simulink model "task1"  (R2021a)
settings: Solver=FixedStepDiscrete  StartTime=0.0  StopTime=10.0  RelTol=1e-3
libraries: simulink x18
settings Model: Creator=NoteBook  LastModifiedBy=NoteBook
settings OptimizationCC: DefaultParameterBehavior=Inlined  EnhancedBackFolding=on  PassReuseOutputArgsAs=Individual arguments  ZeroExternalMemoryAtStartup=off  ZeroInternalMemoryAtStartup=off  OptimizeBlockOrder=speed  DifferentSizesBufferReuse=on  OptimizationCustomize=off  EfficientTunableParamExpr=on
settings DebuggingCC: ParameterTunabilityLossMsg=error
settings SFSimCC: MATLABDynamicMemAlloc=off
settings RTWCC: SystemTargetFile=ert.tlc  GenCodeOnly=on  TemplateMakefile=ert_default_tmf  GenerateReport=on  LaunchReport=on
settings CodeAppCC: ForceParamTrailComments=on  IgnoreCustomStorageClasses=off  OperatorAnnotations=on  SimulinkDataObjDesc=on  SFDataObjDesc=on  InsertBlockDesc=on
settings ERTTargetCC: TargetLangStandard=C99 (ISO)  GenerateSampleERTMain=on  InlinedParameterPlacement=NonHierarchical  ERTCustomFileTemplate=example_file_process.tlc

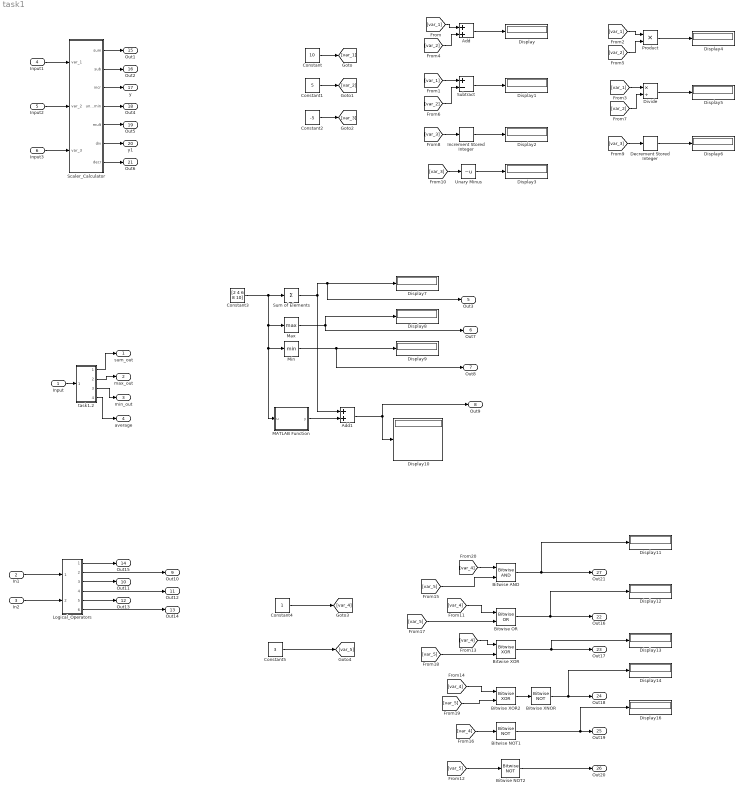
== system task1 ==
  Input : Inport
  In1 : Inport  Port=2
  In2 : Inport  Port=3
  Input1 : Inport  Port=4
  Input2 : Inport  Port=5
  Input3 : Inport  Port=6
  Add : Sum
  Add1 : Sum
  Bitwise AND : simulink/Logic and Bit Operations/Bitwise Operator  logicop=AND  UseBitMask=off  NumInputPorts=2  BitMask=bin2dec('11011001')  BitMaskRealWorld=Stored Integer
  Bitwise NOT1 : simulink/Logic and Bit Operations/Bitwise Operator  logicop=NOT  UseBitMask=off  BitMask=bin2dec('11011001')  BitMaskRealWorld=Stored Integer
  Bitwise NOT2 : simulink/Logic and Bit Operations/Bitwise Operator  logicop=NOT  UseBitMask=off  BitMask=bin2dec('11011001')  BitMaskRealWorld=Stored Integer
  Bitwise OR : simulink/Logic and Bit Operations/Bitwise Operator  logicop=OR  UseBitMask=off  NumInputPorts=2  BitMask=bin2dec('11011001')  BitMaskRealWorld=Stored Integer
  Bitwise XNOR : simulink/Logic and Bit Operations/Bitwise Operator  logicop=NOT  UseBitMask=off  BitMask=bin2dec('11011001')  BitMaskRealWorld=Stored Integer
  Bitwise XOR : simulink/Logic and Bit Operations/Bitwise Operator  logicop=XOR  UseBitMask=off  NumInputPorts=2  BitMask=bin2dec('11011001')  BitMaskRealWorld=Stored Integer
  Bitwise XOR2 : simulink/Logic and Bit Operations/Bitwise Operator  logicop=XOR  UseBitMask=off  NumInputPorts=2  BitMask=bin2dec('11011001')  BitMaskRealWorld=Stored Integer
  Constant : Constant  Value=10
  Constant1 : Constant  Value=5
  Constant2 : Constant  Value=-5
  Constant3 : Constant  Value=[2 4 6 8 10]
  Constant4 : Constant  OutDataTypeStr=uint32
  Constant5 : Constant  Value=3  OutDataTypeStr=uint32
  Decrement Stored Integer : simulink/Additional Math & Discrete/Additional Math: Increment - Decrement/Decrement Stored Integer
      settings: SourceProductBaseCode=SL
  Display{,1..14,16} (16 alike) : Display
  Divide : Product  Inputs=*/
  Increment Stored Integer : simulink/Additional Math & Discrete/Additional Math: Increment - Decrement/Increment Stored Integer
  Logical_Operators : Subsystem
  MATLAB Function : MATLAB Function  TreatAsAtomicUnit=on
  Max : MinMax  Function=max
  Min : MinMax
  Product : Product
  Scaler_Calculator : Subsystem
  Subtract : Sum  Inputs=+-
  Sum of Elements : Sum  Inputs=+
  Unary Minus : UnaryMinus
  task1.2 : Subsystem
  sum_out : Outport
  max_out : Outport  Port=2
  min_out : Outport  Port=3
  average : Outport  Port=4
  Out3 : Outport  Port=5
  Out7 : Outport  Port=6
  Out8 : Outport  Port=7
  Out9 : Outport  Port=8
  Out10 : Outport  Port=9
  Out11 : Outport  Port=10
  Out12 : Outport  Port=11
  Out13 : Outport  Port=12
  Out14 : Outport  Port=13
  Out15 : Outport  Port=14
  Out1 : Outport  Port=15
  Out2 : Outport  Port=16
  y : Outport  Port=17
  Out4 : Outport  Port=18
  Out5 : Outport  Port=19
  y1 : Outport  Port=20
  Out6 : Outport  Port=21
  Out16 : Outport  Port=22
  Out17 : Outport  Port=23
  Out18 : Outport  Port=24
  Out19 : Outport  Port=25
  Out20 : Outport  Port=26
  Out21 : Outport  Port=27
  wires:
  Input/1 -> task1.2/1(In1)
  task1.2/1(Out1) -> sum_out/1
  task1.2/2(Out2) -> max_out/1
  task1.2/3(Out3) -> min_out/1
  task1.2/4(Out4) -> average/1
  Add1/1 -> Out9/1, Display10/1
  Min/1 -> Out8/1, Display9/1
  MATLAB Function/1(y) -> Add1/2
  Max/1 -> Out7/1, Display8/1
  Constant3/1 -> MATLAB Function/1(u), Min/1, Max/1, Sum of Elements/1
  Sum of Elements/1 -> Add1/1, Out3/1, Display7/1
  In1/1 -> Logical_Operators/1(var_1)
  In2/1 -> Logical_Operators/2(var_2)
  Logical_Operators/1(Out1) -> Out15/1
  Logical_Operators/2(Out2) -> Out10/1
  Logical_Operators/3(Out3) -> Out11/1
  Logical_Operators/4(Out4) -> Out12/1
  Logical_Operators/5(Out5) -> Out13/1
  Logical_Operators/6(Out6) -> Out14/1
  [var_1] -> Subtract/1
  [var_3] -> Increment Stored Integer/1
  [var_3] -> Unary Minus/1
  Add/1 -> Display/1
  [var_2] -> Subtract/2
  [var_1] -> Add/1
  Constant1/1 -> [var_2]
  [var_2] -> Add/2
  Scaler_Calculator/5(mult) -> Out5/1
  Scaler_Calculator/7(decr) -> Out6/1
  Unary Minus/1 -> Display3/1
  Constant2/1 -> [var_3]
  Input2/1 -> Scaler_Calculator/2(var_2)
  Input1/1 -> Scaler_Calculator/1(var_1)
  Scaler_Calculator/2(sub) -> Out2/1
  Increment Stored Integer/1 -> Display2/1
  Scaler_Calculator/4(unarymin) -> Out4/1
  Subtract/1 -> Display1/1
  Scaler_Calculator/1(sum) -> Out1/1
  Scaler_Calculator/6(div) -> y1/1
  Scaler_Calculator/3(incr) -> y/1
  Input3/1 -> Scaler_Calculator/3(var_3)
  Constant/1 -> [var_1]
  [var_3] -> Decrement Stored Integer/1
  [var_2] -> Product/2
  [var_1] -> Divide/1
  [var_1] -> Product/1
  [var_2] -> Divide/2
  Divide/1 -> Display5/1
  Decrement Stored Integer/1 -> Display6/1
  Product/1 -> Display4/1
  Constant5/1 -> [var_5]
  [var_5] -> Bitwise OR/2
  [var_5] -> Bitwise XOR2/2
  [var_5] -> Bitwise AND/2
  [var_4] -> Bitwise NOT1/1
  [var_4] -> Bitwise OR/1
  Constant4/1 -> [var_4]
  [var_4] -> Bitwise XOR2/1
  [var_5] -> Bitwise NOT2/1
  Bitwise XOR2/1 -> Bitwise XNOR/1
  [var_4] -> Bitwise XOR/1
  Bitwise NOT1/1 -> Display16/1, Out19/1
  [var_5] -> Bitwise XOR/2
  Bitwise XOR/1 -> Display13/1, Out17/1
  Bitwise NOT2/1 -> Out20/1
  Bitwise OR/1 -> Display12/1, Out16/1
  Bitwise XNOR/1 -> Display14/1, Out18/1
  Bitwise AND/1 -> Display11/1, Out21/1
  [var_4] -> Bitwise AND/1

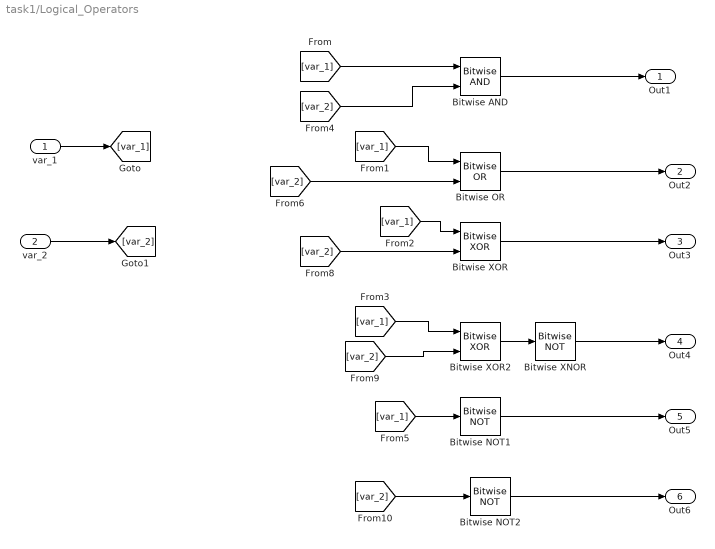
== system task1/Logical_Operators ==
  var_1 : Inport  OutDataTypeStr=uint32
  var_2 : Inport  Port=2  OutDataTypeStr=uint32
  Bitwise AND : simulink/Logic and Bit Operations/Bitwise Operator  logicop=AND  UseBitMask=off  NumInputPorts=2  BitMask=bin2dec('11011001')  BitMaskRealWorld=Stored Integer
  Bitwise NOT1 : simulink/Logic and Bit Operations/Bitwise Operator  logicop=NOT  UseBitMask=off  BitMask=bin2dec('11011001')  BitMaskRealWorld=Stored Integer
  Bitwise NOT2 : simulink/Logic and Bit Operations/Bitwise Operator  logicop=NOT  UseBitMask=off  BitMask=bin2dec('11011001')  BitMaskRealWorld=Stored Integer
  Bitwise OR : simulink/Logic and Bit Operations/Bitwise Operator  logicop=OR  UseBitMask=off  NumInputPorts=2  BitMask=bin2dec('11011001')  BitMaskRealWorld=Stored Integer
  Bitwise XNOR : simulink/Logic and Bit Operations/Bitwise Operator  logicop=NOT  UseBitMask=off  BitMask=bin2dec('11011001')  BitMaskRealWorld=Stored Integer
  Bitwise XOR : simulink/Logic and Bit Operations/Bitwise Operator  logicop=XOR  UseBitMask=off  NumInputPorts=2  BitMask=bin2dec('11011001')  BitMaskRealWorld=Stored Integer
  Bitwise XOR2 : simulink/Logic and Bit Operations/Bitwise Operator  logicop=XOR  UseBitMask=off  NumInputPorts=2  BitMask=bin2dec('11011001')  BitMaskRealWorld=Stored Integer
  Out1 : Outport
  Out2 : Outport  Port=2
  Out3 : Outport  Port=3
  Out4 : Outport  Port=4
  Out5 : Outport  Port=5
  Out6 : Outport  Port=6
  wires:
  Bitwise NOT2/1 -> Out6/1
  Bitwise XOR2/1 -> Bitwise XNOR/1
  Bitwise AND/1 -> Out1/1
  Bitwise XNOR/1 -> Out4/1
  Bitwise OR/1 -> Out2/1
  Bitwise NOT1/1 -> Out5/1
  Bitwise XOR/1 -> Out3/1
  var_1/1 -> [var_1]
  var_2/1 -> [var_2]
  [var_1] -> Bitwise AND/1
  [var_1] -> Bitwise OR/1
  [var_1] -> Bitwise XOR/1
  [var_1] -> Bitwise NOT1/1
  [var_1] -> Bitwise XOR2/1
  [var_2] -> Bitwise AND/2
  [var_2] -> Bitwise NOT2/1
  [var_2] -> Bitwise XOR2/2
  [var_2] -> Bitwise XOR/2
  [var_2] -> Bitwise OR/2

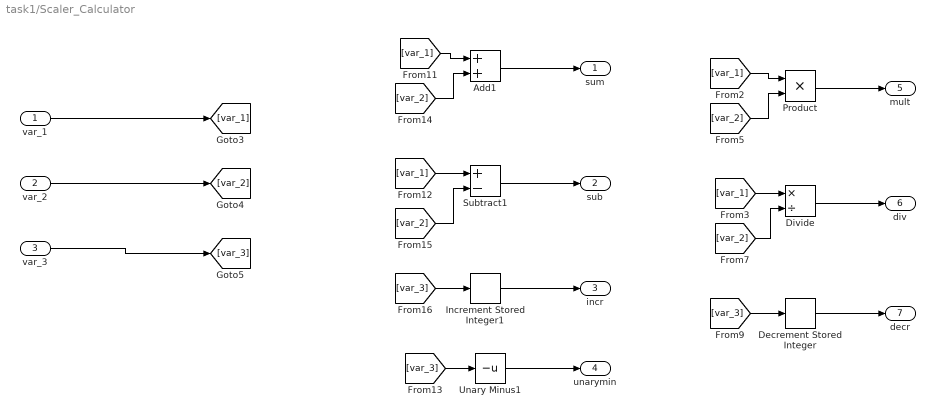
== system task1/Scaler_Calculator ==
  var_1 : Inport
  var_2 : Inport  Port=2
  var_3 : Inport  Port=3
  Add1 : Sum
  Decrement Stored Integer : simulink/Additional Math & Discrete/Additional Math: Increment - Decrement/Decrement Stored Integer
      settings: SourceProductBaseCode=SL
  Divide : Product  Inputs=*/
  Increment Stored Integer1 : simulink/Additional Math & Discrete/Additional Math: Increment - Decrement/Increment Stored Integer
  Product : Product
  Subtract1 : Sum  Inputs=+-
  Unary Minus1 : UnaryMinus
  sum : Outport
  sub : Outport  Port=2
  incr : Outport  Port=3
  unarymin : Outport  Port=4
  mult : Outport  Port=5
  div : Outport  Port=6
  decr : Outport  Port=7
  wires:
  Subtract1/1 -> sub/1
  [var_3] -> Increment Stored Integer1/1
  [var_2] -> Add1/2
  Increment Stored Integer1/1 -> incr/1
  [var_1] -> Add1/1
  [var_2] -> Subtract1/2
  [var_3] -> Unary Minus1/1
  [var_1] -> Subtract1/1
  var_3/1 -> [var_3]
  var_2/1 -> [var_2]
  Unary Minus1/1 -> unarymin/1
  var_1/1 -> [var_1]
  Add1/1 -> sum/1
  [var_2] -> Product/2
  [var_3] -> Decrement Stored Integer/1
  [var_1] -> Product/1
  [var_2] -> Divide/2
  [var_1] -> Divide/1
  Decrement Stored Integer/1 -> decr/1
  Product/1 -> mult/1
  Divide/1 -> div/1

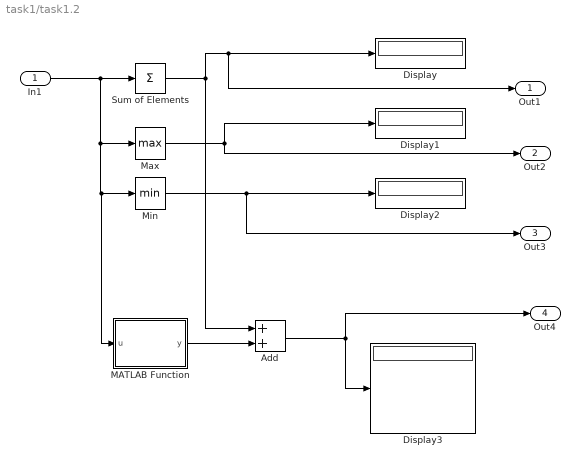
== system task1/task1.2 ==
  In1 : Inport
  Add : Sum
  Display{,1..3} (4 alike) : Display
  MATLAB Function : MATLAB Function  TreatAsAtomicUnit=on
  Max : MinMax  Function=max
  Min : MinMax
  Sum of Elements : Sum  Inputs=+
  Out1 : Outport
  Out2 : Outport  Port=2
  Out3 : Outport  Port=3
  Out4 : Outport  Port=4
  wires:
  Sum of Elements/1 -> Add/1, Out1/1, Display/1
  In1/1 -> MATLAB Function/1(u), Min/1, Max/1, Sum of Elements/1
  Min/1 -> Out3/1, Display2/1
  Max/1 -> Out2/1, Display1/1
  Add/1 -> Out4/1, Display3/1
  MATLAB Function/1(y) -> Add/2

== matlab function task1/task1.2/MATLAB Function ==
  data: u input; y output
function y = fcn(u)

y = u;

== matlab function task1/MATLAB Function ==
  data: u input; y output
function y = fcn(u)

y = u;
